simulink model "Simscape_Language_Springs_7"  (R2014a)
settings: Solver=ode23t  StartTime=0.0  StopTime=15  RelTol=1e-3
InitFcn:
  | warning off Simulink:SL_MatchingFromNotFound
  | m=1;
  | b=1;
  | k=1;
libraries: fl_lib x14, nesl_utility x6, CustomSprings_lib x2
Description:
  | Copyright 2014 The MathWorks, Inc.
settings Model: Creator=tegel  LastModifiedBy=smiller
settings DataIOCC: SignalLoggingSaveFormat=ModelDataLogs
settings OptimizationCC: ExpressionDepthLimit=2147483647  InitFltsAndDblsToZero=on
settings DebuggingCC: SaveWithParameterizedLinksMsg=none  UnderspecifiedInitializationDetection=Classic  FcnCallInpInsideContextMsg=UseLocalSettings  StateNameClashWarn=warning
settings GRTTargetCC: TargetFcnLib=ansi_tfl_tmw.mat  CombineOutputUpdateFcns=off  GRTInterface=on

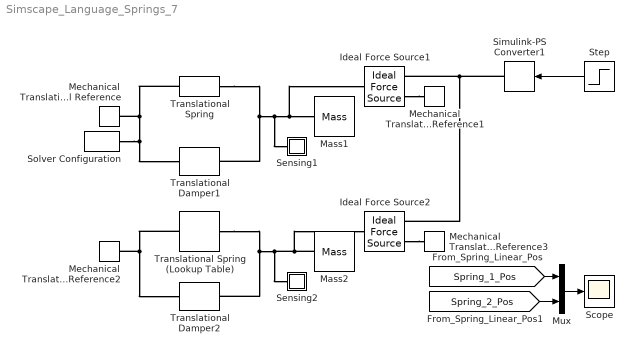
== system Simscape_Language_Springs_7 ==
  Ideal Force Source1 : fl_lib/Mechanical/Mechanical Sources/Ideal Force Source
  Ideal Force Source2 : fl_lib/Mechanical/Mechanical Sources/Ideal Force Source
  Mass1 : fl_lib/Mechanical/Translational Elements/Mass  mass=m kg  v_specify=on  v_priority=High  v=0 m/s  f_specify=off  f_priority=High  f=0 N
  Mass2 : fl_lib/Mechanical/Translational Elements/Mass  mass=m kg  v_specify=on  v_priority=High  v=0 m/s  f_specify=off  f_priority=High  f=0 N
  Mechanical Translational Reference{,1..3} (4 alike) : fl_lib/Mechanical/Translational Elements/Mechanical Translational Reference
  Mux : Mux  Inputs=2
  Scope : Scope
      settings: TimeRange=15  YMin=0  YMax=2.5
  Sensing1 : Subsystem
  Sensing2 : Subsystem
  Simulink-PS Converter1 : nesl_utility/Simulink-PS Converter  PhysicalDomain=network_engine_domain  SubClassName=ps_input  LeftPortType=input  RightPortType=output  PseudoPeriodic=off  Frequencies=[]  NoiseDistribution=none  NoiseParameters=[]  Unit=1  AffineConversion=off  InputFiltering=off  SimscapeFilterOrder=1  InputFilterTimeConstant=.001  UdotUserProvided=0
  Solver Configuration : nesl_utility/Solver Configuration  PhysicalDomain=network_engine_domain  SubClassName=solver  LeftPortType=input  RightPortType=generic  Accelerate=off  Tones=[]  Harmonics=[]  SimulateNoise=off  Profile=off  UseLocalSampling=off  EnableSwitchedLinearOptims=on  FrequencyDomain=off  UseCCode=off  RelTol=0.001  AbsTol=1e-06  MinStep=1e-09  ToWorkspace=off  DoDC=off  ResidualTolerance=1e-9  UseLocalSolver=off  LocalSolverChoice=NE_BACKWARD_EULER_ADVANCER  LocalSolverSampleTime=.001  DoFixedCost=off  MaxNonlinIter=12  MaxModeIter=2  LinearAlgebra=Sparse  DelaysMemoryBudget=1024  AutomaticFiltering=on  FilteringTimeConstant=0.001
  Step : Step  After=2  SampleTime=0
  Translational Damper1 : fl_lib/Mechanical/Translational Elements/Translational Damper  D=b N/(m/s)  v_specify=off  v_priority=High  v=0 m/s  f_specify=off  f_priority=High  f=0 N
  Translational Damper2 : fl_lib/Mechanical/Translational Elements/Translational Damper  D=b N/(m/s)  v_specify=off  v_priority=High  v=0 m/s  f_specify=off  f_priority=High  f=0 N
  Translational Spring : CustomSprings_lib/Translational Spring  k=1 N/m  v_specify=off  v_priority=High  v=0 m/s  f_specify=off  f_priority=High  f=0 N  x_specify=off  x_priority=High  x=0 m
  Translational Spring (Lookup Table) : CustomSprings_lib/Translational Spring (Lookup Table)  xd=[ -4 -3 -2 -1 0 1 2 3 4 ] m  kd=[1e+6 8 4 2 0 2 4 8 1e+6] N/m  v_specify=off  v_priority=High  v=0 m/s  f_specify=off  f_priority=High  f=0 N  x_specify=off  x_priority=High  x=0 m  k_specify=off  k_priority=High  k=0 N/m
  wires:
  Mux/1 -> Scope/1
  [Spring_1_Pos] -> Mux/1
  [Spring_2_Pos] -> Mux/2
  Step/1 -> Simulink-PS Converter1/1
  connections:
  Simulink-PS Converter1/RConn1 -- Ideal Force Source1/RConn1 -- Ideal Force Source2/RConn1
  Ideal Force Source1/RConn2 -- Mechanical Translational Reference1/LConn1
  Translational Spring/LConn1 -- Mechanical Translational Reference/LConn1 -- Translational Damper1/RConn1 -- Solver Configuration/RConn1
  Translational Spring/RConn1 -- Translational Damper1/LConn1 -- Sensing1/LConn1 -- Mass1/LConn1 -- Ideal Force Source1/LConn1
  Translational Spring (Lookup Table)/LConn1 -- Mechanical Translational Reference2/LConn1 -- Translational Damper2/RConn1
  Translational Spring (Lookup Table)/RConn1 -- Translational Damper2/LConn1 -- Sensing2/LConn1 -- Mass2/LConn1 -- Ideal Force Source2/LConn1
  Ideal Force Source2/RConn2 -- Mechanical Translational Reference3/LConn1

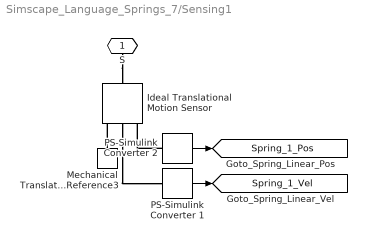
== system Simscape_Language_Springs_7/Sensing1 ==
  Ideal Translational Motion Sensor : fl_lib/Mechanical/Mechanical Sensors/Ideal Translational Motion Sensor  offset=0 m
  Mechanical Translational Reference3 : fl_lib/Mechanical/Translational Elements/Mechanical Translational Reference
  PS-Simulink Converter 1 : nesl_utility/PS-Simulink Converter  PhysicalDomain=network_engine_domain  SubClassName=ps_output  LeftPortType=input  RightPortType=output  PseudoPeriodic=off  Frequencies=[]  Unit=1  AffineConversion=off
  PS-Simulink Converter 2 : nesl_utility/PS-Simulink Converter  PhysicalDomain=network_engine_domain  SubClassName=ps_output  LeftPortType=input  RightPortType=output  PseudoPeriodic=off  Frequencies=[]  Unit=1  AffineConversion=off
  S : PMIOPort  Port=1  Side=Left
  tag scope: Spring_1_Pos=global, Spring_1_Vel=global
  wires:
  PS-Simulink Converter 2/1 -> [Spring_1_Pos]
  PS-Simulink Converter 1/1 -> [Spring_1_Vel]
  connections:
  S/RConn1 -- Ideal Translational Motion Sensor/LConn1
  Mechanical Translational Reference3/LConn1 -- Ideal Translational Motion Sensor/RConn1
  Ideal Translational Motion Sensor/RConn2 -- PS-Simulink Converter 1/LConn1
  PS-Simulink Converter 2/LConn1 -- Ideal Translational Motion Sensor/RConn3

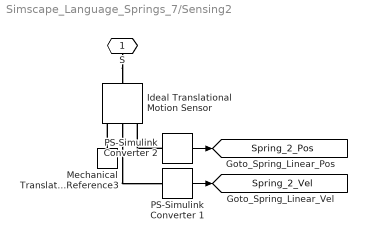
== system Simscape_Language_Springs_7/Sensing2 ==
  Ideal Translational Motion Sensor : fl_lib/Mechanical/Mechanical Sensors/Ideal Translational Motion Sensor  offset=0 m
  Mechanical Translational Reference3 : fl_lib/Mechanical/Translational Elements/Mechanical Translational Reference
  PS-Simulink Converter 1 : nesl_utility/PS-Simulink Converter  PhysicalDomain=network_engine_domain  SubClassName=ps_output  LeftPortType=input  RightPortType=output  PseudoPeriodic=off  Frequencies=[]  Unit=1  AffineConversion=off
  PS-Simulink Converter 2 : nesl_utility/PS-Simulink Converter  PhysicalDomain=network_engine_domain  SubClassName=ps_output  LeftPortType=input  RightPortType=output  PseudoPeriodic=off  Frequencies=[]  Unit=1  AffineConversion=off
  S : PMIOPort  Port=1  Side=Left
  tag scope: Spring_2_Pos=global, Spring_2_Vel=global
  wires:
  PS-Simulink Converter 1/1 -> [Spring_2_Vel]
  PS-Simulink Converter 2/1 -> [Spring_2_Pos]
  connections:
  PS-Simulink Converter 2/LConn1 -- Ideal Translational Motion Sensor/RConn3
  Ideal Translational Motion Sensor/RConn2 -- PS-Simulink Converter 1/LConn1
  Mechanical Translational Reference3/LConn1 -- Ideal Translational Motion Sensor/RConn1
  S/RConn1 -- Ideal Translational Motion Sensor/LConn1
